simulink model "mae_free"  (R2021b)
settings: Solver=VariableStepAuto  StartTime=0.0  StopTime=10  MaxStep=0.005  RelTol=1e-3  AbsTol=1e-3  EnableMultiTasking=on
PostLoadFcn:
  | m = 3.600;     % kg
  | k = 400;    % N/m
  | b = 10;      % Ns/m
libraries: fl_lib x6, nesl_utility x3, simulink x1
CloseFcn:
  | try,close(h1_ssc_mass_spring_damper_sl_dbl),end
  | clear h1_ssc_mass_spring_damper_sl_dbl
  | 
  | clear simlog_ssc_mass_spring_damper_sl_dbl
  | clear logsout_ssc_mass_spring_damper_sl_dbl
Description:
  | Double Mass-Spring-Damper in Simulink(R) and Simscape(TM)
settings Model: Creator=The MathWorks, Inc.  LastModifiedBy=Admin
settings SolverCC: AutoScaleAbsTol=off  AlgebraicLoopSolver=TrustRegion
settings DataIOCC: SaveFormat=Array  ReturnWorkspaceOutputs=off  SignalLoggingName=logsout_ssc_mass_spring_damper_sl_dbl
settings OptimizationCC: LifeSpan=inf
settings DebuggingCC: SolverPrmCheckMsg=warning  AllowSymbolicDim=off  PregeneratedLibrarySubsystemCodeDiagnostic=none  SFUnexpectedBacktrackingDiag=warning  SFNoUnconditionalDefaultTransitionDiag=warning  SFExecutionAtInitializationDiag=none  SFMachineParentedDataDiag=warning  ArithmeticOperatorsInVariantConditions=warning
settings HardwareCC: ProdBitPerPointer=32  ProdBitPerSizeT=32  ProdBitPerPtrDiffT=32  ProdLargestAtomicFloat=None  ProdIntDivRoundTo=Undefined  ProdEndianess=Unspecified  ProdWordSize=32  ProdHWDeviceType=32-bit Generic
settings ModelReferenceCC: PropagateSignalLabelsOutOfModel=off
settings SFSimCC: SimUseLocalCustomCode=off  CustomCodeUndefinedFunction=UseInterfaceOnly
settings RTWCC: RTWUseLocalCustomCode=off
settings CodeAppCC: StateflowObjectComments=on
settings GRTTargetCC: TargetLangStandard=C89/C90 (ANSI)
settings ConfigComp: CovMetricSettings=dw  CovSaveCumulativeToWorkspaceVar=on  CovSaveSingleToWorkspaceVar=on  CovExternalEMLEnable=off  CovSFcnEnable=off
settings SimscapeCC: SimscapeLogType=all  SimscapeLogSimulationStatistics=on  SimscapeLogName=simlog_ssc_mass_spring_damper_sl_dbl  SimscapeLogDataHistory=10000

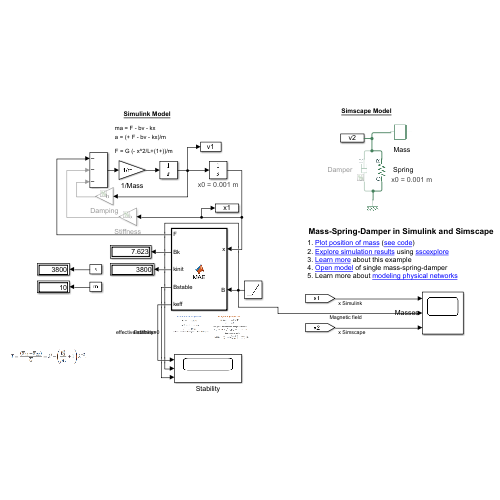
[thumbnail: Simulink's stored preview of the top-level diagram]
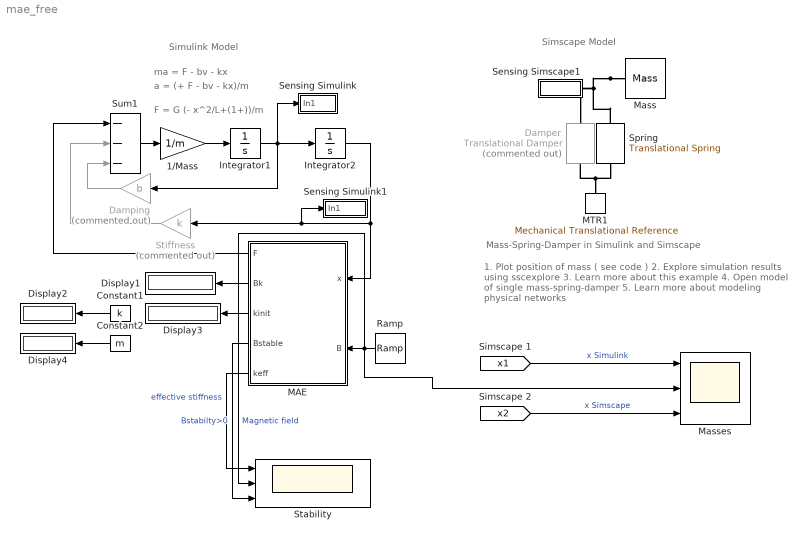
== system mae_free ==
  note: a = (+ F - bv - kx)/m
  note: 1. Plot position of mass ( see code )
      | 2. Explore simulation results using sscexplore
      | 3. Learn more about this example
      | 4. Open model of single mass-spring-damper
      | 5. Learn more about modeling physical networks
  note: Mass-Spring-Damper in Simulink and Simscape
  note: Simulink Model
  note: Simscape Model
  note: ma = F - bv - kx
  note: F = G (- x^2/L+(1+))/m
  1/Mass : Gain  Gain=1/m  SaturateOnIntegerOverflow=on  OutDataTypeStr=Inherit: Same as input  ParamDataTypeStr=Inherit: Same as input
  Constant1 : Constant  Value=k
  Constant2 : Constant  Value=m
  Damper : fl_lib/Mechanical/Translational Elements/Translational Damper  Commented=on  D=b N/(m/s)  v_specify=off  v_priority=High  v=0 m/s  v_nominal_specify=off  v_nominal_unit=m/s  v_nominal_value=1  f_specify=off  f_priority=High  f=0 N  f_nominal_specify=off  f_nominal_unit=N  f_nominal_value=1
  Damping : Gain  Commented=on  Gain=b  SaturateOnIntegerOverflow=on  OutDataTypeStr=Inherit: Same as input  ParamDataTypeStr=Inherit: Same as input
  Display{1..4} (4 alike) : Display
  Integrator1 : Integrator
  Integrator2 : Integrator  InitialCondition=0.001
      settings: AttributesFormatString=x0 = %<InitialCondition> m
  MAE : MATLAB Function  TreatAsAtomicUnit=on
  MTR1 : fl_lib/Mechanical/Translational Elements/Mechanical Translational Reference
  Mass : fl_lib/Mechanical/Translational Elements/Mass  mass=m kg  num_ports=foundation.enum.numPorts2.one  v_specify=off  v_priority=High  v=0 m/s  v_nominal_specify=off  v_nominal_unit=m/s  v_nominal_value=1  f_specify=off  f_priority=High  f=0 N  f_nominal_specify=off  f_nominal_unit=N  f_nominal_value=1
  Masses : Scope  NumInputPorts=3
  Ramp : simulink/Sources/Ramp  slope=0.1  start=0  InitialOutput=0
  Sensing Simscape1 : Subsystem
      mask Display: disp('v2')
  Sensing Simulink : Subsystem
      mask Display: disp('v1')
  Sensing Simulink1 : Subsystem
      mask Display: disp('x1')
  Spring : fl_lib/Mechanical/Translational Elements/Translational Spring  spr_rate=k N/m  v_specify=off  v_priority=High  v=0 m/s  v_nominal_specify=off  v_nominal_unit=m/s  v_nominal_value=1  f_specify=off  f_priority=High  f=0 N  f_nominal_specify=off  f_nominal_unit=N  f_nominal_value=1  x_specify=on  x_priority=High  x=0.001 m  x_nominal_specify=off  x_nominal_unit=m  x_nominal_value=1
      settings: AttributesFormatString=x0 = %<x> %<x_unit>
  Stability : Scope  NumInputPorts=3
  Stiffness : Gain  Commented=on  Gain=k  SaturateOnIntegerOverflow=on  OutDataTypeStr=Inherit: Same as input  ParamDataTypeStr=Inherit: Same as input
  Sum1 : Sum  Inputs=---  InputSameDT=on  SaturateOnIntegerOverflow=on  OutDataTypeStr=Inherit: Same as first input
  wires:
  1/Mass/1 -> Integrator1/1
  Sum1/1 -> 1/Mass/1
  Damping/1 -> Sum1/3
  Stiffness/1 -> Sum1/2
  Integrator2/1 -> Sensing Simulink1/1(In1), Stiffness/1, MAE/1(x)
  Integrator1/1 -> Sensing Simulink/1(In1), Integrator2/1, Damping/1
  MAE/1(F) -> Sum1/1
  Ramp/1 -> Masses/2, Stability/2, MAE/2(B)  "Magnetic field"
  MAE/2(Bk) -> Display1/1
  Constant1/1 -> Display2/1
  [x2] -> Masses/3  "x Simscape"
  [x1] -> Masses/1  "x Simulink"
  MAE/4(Bstable) -> Stability/3  "Bstabilty>0"
  MAE/3(kinit) -> Display3/1
  Constant2/1 -> Display4/1
  MAE/5(keff) -> Stability/1  "effective stiffness"
  connections:
  Spring/RConn1 -- Damper/RConn1 -- MTR1/LConn1
  Mass/LConn1 -- Sensing Simscape1/LConn1 -- Spring/LConn1 -- Damper/LConn1

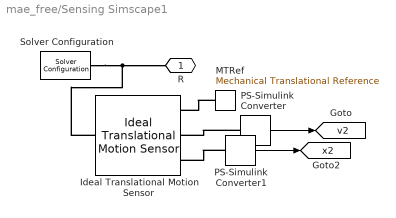
== system mae_free/Sensing Simscape1 ==
  Ideal Translational Motion Sensor : fl_lib/Mechanical/Mechanical Sensors/Ideal Translational Motion Sensor  offset=1e-3 m
  MTRef : fl_lib/Mechanical/Translational Elements/Mechanical Translational Reference
  PS-Simulink Converter : nesl_utility/PS-Simulink Converter  PhysicalDomain=network_engine_domain  SubClassName=ps_output  LeftPortType=input  RightPortType=output  PseudoPeriodic=off  Frequencies=[]  Unit=1  AffineConversion=off
      settings: SourceProductBaseCode=PW,SS
  PS-Simulink Converter1 : nesl_utility/PS-Simulink Converter  PhysicalDomain=network_engine_domain  SubClassName=ps_output  LeftPortType=input  RightPortType=output  PseudoPeriodic=off  Frequencies=[]  Unit=1  AffineConversion=off
      settings: SourceProductBaseCode=PW,SS
  Solver Configuration : nesl_utility/Solver Configuration  PhysicalDomain=network_engine_domain  SubClassName=solver  LeftPortType=input  RightPortType=generic  Tones=[]  Harmonics=[]  SimulateNoise=off  Profile=off  UseLocalSampling=off  EnableSwitchedLinearOptims=on  FrequencyDomain=off  UseCCode=off  RelTol=0.001  AbsTol=1e-06  MinStep=1e-09  ToWorkspace=off  RevertToSquareIcSolve=off  NumHomotopyIterations=100  PhasorMode=off  PhasorModeNumHarmonics=1  DoDC=off  ResidualTolerance=1e-9  UseLocalSolver=off  LocalSolverChoice=NE_BACKWARD_EULER_ADVANCER  LocalSolverSampleTime=.001  DoFixedCost=off  MaxNonlinIter=12  MaxModeIter=2  ComputeImpulses=off  ImpulseIterations=2  LinearAlgebra=auto  EquationFormulation=NE_TIME_EF  DelaysMemoryBudget=1024  AutomaticFiltering=on  FilteringTimeConstant=0.001  PartitionStorageMethod=AS_NEEDED  PartitionMemoryBudget=1024  PartitionMethod=FAST
      settings: SourceProductBaseCode=PW,SS
  R : PMIOPort  Side=Left
  tag scope: v2=global, x2=global
  wires:
  PS-Simulink Converter/1 -> [v2]
  PS-Simulink Converter1/1 -> [x2]
  connections:
  MTRef/LConn1 -- Ideal Translational Motion Sensor/RConn1
  PS-Simulink Converter/LConn1 -- Ideal Translational Motion Sensor/RConn2
  Ideal Translational Motion Sensor/LConn1 -- Solver Configuration/RConn1 -- R/RConn1
  PS-Simulink Converter1/LConn1 -- Ideal Translational Motion Sensor/RConn3

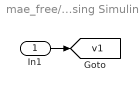
== system mae_free/Sensing Simulink ==
  In1 : Inport
  tag scope: v1=global
  wires:
  In1/1 -> [v1]

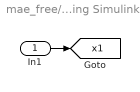
== system mae_free/Sensing Simulink1 ==
  In1 : Inport
  tag scope: x1=global
  wires:
  In1/1 -> [x1]

== matlab function mae_free/MAE ==
  data: x input; B input; F output; Bk output; kinit output; Bstable output; keff output
function [F,Bk,kinit,Bstable,keff] = MAE(x,B)

G1 = 50*1e3;    c1 = 0.9;       mu1 = 1;                                
G2 = 500*1e3;   c2 = 0.1;       mu2 = 10;                               

mu0 = 1.25663706 * 1e-6;        L0 = 0.01;
Gbar = G1*c1 + G2*c2;           mubar = mu0*(mu1*c1 + mu2*c2);   
Gcap = 1/(c1/G1 + c2/G2);       mucap = mu0/(c1/mu1 + c2/mu2);

A = L0*L0;

ld = 1 + x/L0;                   Bk =  B^2/(mucap*Gbar);
kinit = A*Gbar*(2 + 2)/L0;
keff = A*Gbar*2*(ld + 1/ld^3 + Bk/ld^3)/L0;

F = A*Gbar*(ld^2 - 1/ld^2 - Bk/ld^2);
Bstable = sqrt((ld^4-1+Gcap/Gbar)*(mucap*Gbar)/(1-mucap/mubar)) - B;

end
